simulink model "pt1_sin_waves_saturation"  (R2019a)
settings: Solver=ode4  StartTime=0.0  StopTime=1  FixedStep=0.001  RelTol=1e-3
settings Model: Creator=guima  LastModifiedBy=guima

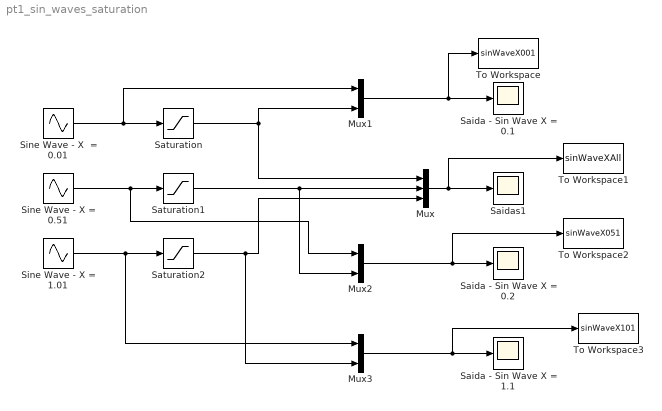
== system pt1_sin_waves_saturation ==
  Mux : Mux  Inputs=3
  Mux1 : Mux  Inputs=2
  Mux2 : Mux  Inputs=2
  Mux3 : Mux  Inputs=2
  Saida - Sin Wave X = 0.1 : Scope
  Saida - Sin Wave X = 0.2 : Scope
  Saida - Sin Wave X = 1.1 : Scope
  Saidas1 : Scope
  Saturation : Saturate  UpperLimit=0.1  LowerLimit=-0.1
  Saturation1 : Saturate  UpperLimit=0.1  LowerLimit=-0.1
  Saturation2 : Saturate  UpperLimit=0.1  LowerLimit=-0.1
  Sine Wave - X  = 0.01 : Sin  Amplitude=0.01  Frequency=2*pi  SampleTime=0
  Sine Wave - X = 0.51 : Sin  Amplitude=0.51  Frequency=2*pi  SampleTime=0
  Sine Wave - X = 1.01 : Sin  Amplitude=1.01  Frequency=2*pi  SampleTime=0
  To Workspace : ToWorkspace  VariableName=sinWaveX001  SaveFormat=Structure With Time  SampleTime=-1
  To Workspace1 : ToWorkspace  VariableName=sinWaveXAll  SaveFormat=Structure With Time  SampleTime=-1
  To Workspace2 : ToWorkspace  VariableName=sinWaveX051  SaveFormat=Structure With Time  SampleTime=-1
  To Workspace3 : ToWorkspace  VariableName=sinWaveX101  SaveFormat=Structure With Time  SampleTime=-1
  wires:
  Sine Wave - X = 0.51/1 -> Saturation1/1, Mux2/1
  Sine Wave - X  = 0.01/1 -> Saturation/1, Mux1/1
  Sine Wave - X = 1.01/1 -> Saturation2/1, Mux3/1
  Saturation1/1 -> Mux2/2, Mux/2
  Saturation2/1 -> Mux3/2, Mux/3
  Saturation/1 -> Mux/1, Mux1/2
  Mux/1 -> To Workspace1/1, Saidas1/1
  Mux3/1 -> To Workspace3/1, Saida - Sin Wave X = 1.1/1
  Mux1/1 -> To Workspace/1, Saida - Sin Wave X = 0.1/1
  Mux2/1 -> To Workspace2/1, Saida - Sin Wave X = 0.2/1
